simulink model "Fig1718"  (R2023b)
settings: Solver=ode1  StartTime=0.0  StopTime=32100  FixedStep=1  RelTol=1e-3
settings Model: Creator=orlandojorquera  LastModifiedBy=evogel

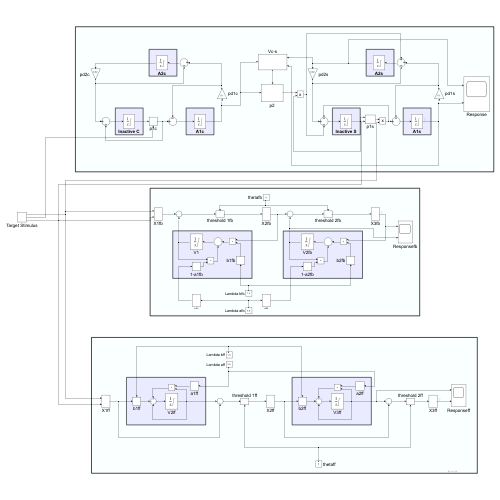
[thumbnail: Simulink's stored preview of the top-level diagram]
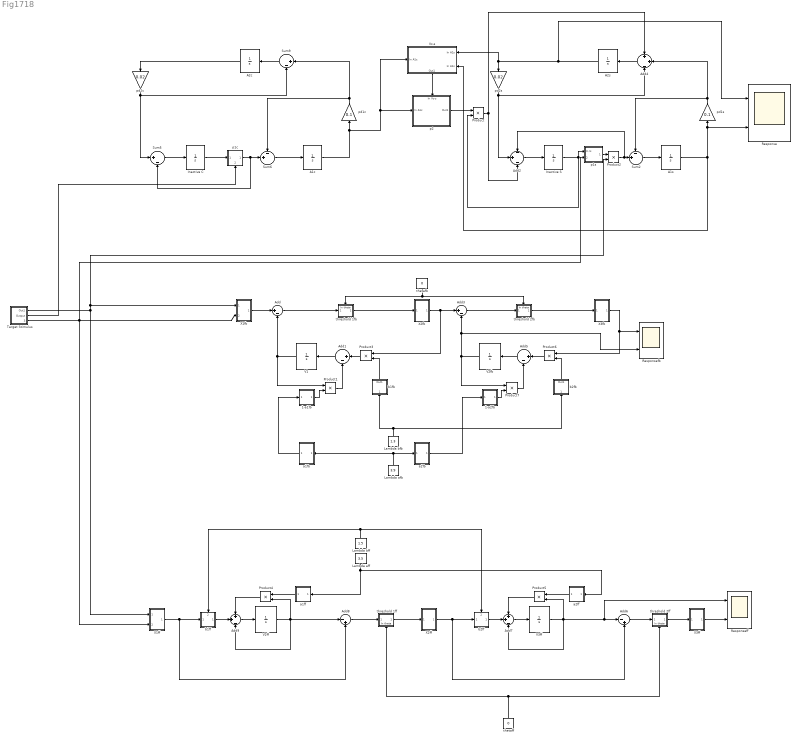
== system Fig1718 ==
  1-a1fb : Subsystem
  1-a2fb : Subsystem
  A1c : Integrator  LimitOutput=on  LowerSaturationLimit=0
  A1s : Integrator  LimitOutput=on  LowerSaturationLimit=0
  A2c : Integrator  LimitOutput=on  LowerSaturationLimit=0
  A2s : Integrator  LimitOutput=on  LowerSaturationLimit=0
  Add{,1,3,5} (4 alike) : Sum  Inputs=|+-
  Add2 : Sum  Inputs=-|+|-
  Add4 : Sum  Inputs=+|+|-
  Add6 : Sum  Inputs=|-+
  Add7 : Sum  Inputs=+|+|-
  Add8 : Sum  Inputs=|-+
  Add9 : Sum  Inputs=+|+|-
  Inactive C : Integrator  InitialCondition=1  LimitOutput=on  LowerSaturationLimit=0
  Inactive S : Integrator  InitialCondition=1  LimitOutput=on  LowerSaturationLimit=0
  Lambda afb : Constant  Value=3.9
  Lambda aff : Constant  Value=3.5
  Lambda bfb : Constant  Value=1.3
  Lambda bff : Constant  Value=1.5
  Product{,1..7} (8 alike) : Product
  Response : Scope  NumInputPorts=2
  Responsefb : Scope  NumInputPorts=2
  Responseff : Scope  NumInputPorts=2
  Sum2 : Sum  Inputs=-+|
  Sum5 : Sum  Inputs=|+-
  Sum6 : Sum  Inputs=-+|
  Sum9 : Sum  Inputs=|+-
  Target Stimulus : Subsystem
  V1 : Integrator  LimitOutput=on
  V2fb : Integrator  LimitOutput=on
  V2ff : Integrator  LimitOutput=on
  V3ff : Integrator  LimitOutput=on
  Vc-s : Subsystem
      settings: PortSchema="{\"entries\":[{\"content\":{\"sides\":[{\"content\":{\"connectorIds\":[\"In1\"]},\"type\":\"ConnectorPlacement.EquallySpacedRectSide\",\"uuid\":\"b09f05bd-5603-47fe-a5ad-d7d6b3dc0c8e\"},{\"content\":{\"connectorIds\":[\"In2\",\"In3\"],\"side\":\"RIGHT\"},\"type\":\"ConnectorPlacement.EquallySpacedRectSide\",\"uuid\":\"d47795f3-6d8c-4c23-a554-34b772022c1b\"},{\"content\":{\"side\":\"TOP\"},\"type\":\"ConnectorPlacement.EquallySpacedRectSide\",\"uuid\":\"e48eddfd-d331-425c-b357-ebbea553df38\"},{\"content\":{\"connectorIds\":[\"Out1\"],\"side\":\"BOTTOM\"},\"type\":\"ConnectorPlacement.EquallySpacedRectSide\",\"uuid\":\"833a9385-f8e7-4f69-9c09-473a519a1ef8\"}]},\"type\":\"ConnectorPlacement.EquallySpacedConnector\",\"uuid\":\"43dd1673-4710-4827-90f7-71f5e88827f7\"}],\"packageUris\":[\"http://schema.mathworks.com/mf0/Connector/R2020b\"],\"version\":\"1.0\"}"
  X1fb : Subsystem
  X1ff : Subsystem
  X2fb : Subsystem
  X2ff : Subsystem
  X3fb : Subsystem
  X3ff : Subsystem
  a1fb : Subsystem
  a1ff : Subsystem
  a2fb : Subsystem
  a2ff : Subsystem
  b1fb : Subsystem
  b1ff : Subsystem
      settings: PortSchema="{\"entries\":[{\"content\":{\"sides\":[{\"content\":{\"connectorIds\":[\"In1\"]},\"type\":\"ConnectorPlacement.EquallySpacedRectSide\",\"uuid\":\"5cafafed-fb19-4a9c-b5ff-e68617ed0211\"},{\"content\":{\"connectorIds\":[\"Out1\"],\"side\":\"RIGHT\"},\"type\":\"ConnectorPlacement.EquallySpacedRectSide\",\"uuid\":\"a77dc629-061a-4bf4-a80e-b7ca5c1ed4cd\"},{\"content\":{\"connectorIds\":[\"In2\"],\"side\":\"TOP\"},\"type\":\"ConnectorPlacement.EquallySpacedRectSide\",\"uuid\":\"07c5d7ad-6053-41a5-acdb-1c90061be6dc\"}]},\"type\":\"ConnectorPlacement.EquallySpacedConnector\",\"uuid\":\"79321a58-c601-4809-afd2-d30de13f135a\"}],\"packageUris\":[\"http://schema.mathworks.com/mf0/Connector/R2020b\"],\"version\":\"1.0\"}"
  b2fb : Subsystem
  b2ff : Subsystem
      settings: PortSchema="{\"entries\":[{\"content\":{\"sides\":[{\"content\":{\"connectorIds\":[\"In1\"]},\"type\":\"ConnectorPlacement.EquallySpacedRectSide\",\"uuid\":\"5cafafed-fb19-4a9c-b5ff-e68617ed0211\"},{\"content\":{\"connectorIds\":[\"Out1\"],\"side\":\"RIGHT\"},\"type\":\"ConnectorPlacement.EquallySpacedRectSide\",\"uuid\":\"a77dc629-061a-4bf4-a80e-b7ca5c1ed4cd\"},{\"content\":{\"connectorIds\":[\"In2\"],\"side\":\"TOP\"},\"type\":\"ConnectorPlacement.EquallySpacedRectSide\",\"uuid\":\"07c5d7ad-6053-41a5-acdb-1c90061be6dc\"}]},\"type\":\"ConnectorPlacement.EquallySpacedConnector\",\"uuid\":\"79321a58-c601-4809-afd2-d30de13f135a\"}],\"packageUris\":[\"http://schema.mathworks.com/mf0/Connector/R2020b\"],\"version\":\"1.0\"}"
  p1c : Subsystem
      settings: PortSchema="{\"entries\":[{\"content\":{\"sides\":[{\"content\":{\"connectorIds\":[\"In1\"]},\"type\":\"ConnectorPlacement.EquallySpacedRectSide\",\"uuid\":\"f7a9d23e-8fc7-4308-b994-1d41de704125\"},{\"content\":{\"connectorIds\":[\"Out1\"],\"side\":\"RIGHT\"},\"type\":\"ConnectorPlacement.EquallySpacedRectSide\",\"uuid\":\"dfc0205e-3a52-4ff6-ace9-e9ebe39396a1\"},{\"content\":{\"side\":\"TOP\"},\"type\":\"ConnectorPlacement.EquallySpacedRectSide\",\"uuid\":\"7914cb48-207a-4343-a956-bdfd7fe7ecdd\"},{\"content\":{\"connectorIds\":[\"In2\"],\"side\":\"BOTTOM\"},\"type\":\"ConnectorPlacement.EquallySpacedRectSide\",\"uuid\":\"56101731-0c9e-48a4-bdfd-b7c152720658\"}]},\"type\":\"ConnectorPlacement.EquallySpacedConnector\",\"uuid\":\"a86337d0-cbcf-4677-827f-1f8aa0c41de3\"}],\"packageUris\":[\"http://schema.mathworks.com/mf0/Connector/R2020b\"],\"version\":\"1.0\"}"
  p1s : Subsystem
  p2 : Subsystem
      settings: PortSchema="{\"entries\":[{\"content\":{\"sides\":[{\"content\":{\"connectorIds\":[\"In1\"]},\"type\":\"ConnectorPlacement.EquallySpacedRectSide\",\"uuid\":\"e5de33b1-e289-4f06-b16e-f6995d6ff18d\"},{\"content\":{\"connectorIds\":[\"Out1\"],\"side\":\"RIGHT\"},\"type\":\"ConnectorPlacement.EquallySpacedRectSide\",\"uuid\":\"bf82b542-ee2f-4a07-ac72-0e3e2437644b\"},{\"content\":{\"connectorIds\":[\"In2\"],\"side\":\"TOP\"},\"type\":\"ConnectorPlacement.EquallySpacedRectSide\",\"uuid\":\"dbd75b9a-fc8b-4088-9d34-f07ad0492047\"}]},\"type\":\"ConnectorPlacement.EquallySpacedConnector\",\"uuid\":\"24fb73df-5fe4-4caa-a2a9-0eaf37dbdd75\"}],\"packageUris\":[\"http://schema.mathworks.com/mf0/Connector/R2020b\"],\"version\":\"1.0\"}"
  pd1c : Gain  Gain=0.1
  pd1s : Gain  Gain=0.1
  pd2c : Gain  Gain=0.02
  pd2s : Gain  Gain=0.02
  thetafb : Constant  Value=0
  thetaff : Constant  Value=0
  threshold 1fb : Subsystem
      settings: PortSchema="{\"entries\":[{\"content\":{\"sides\":[{\"content\":{\"connectorIds\":[\"In1\"]},\"type\":\"ConnectorPlacement.EquallySpacedRectSide\",\"uuid\":\"df45c11a-cbfd-46b0-9931-ccf6bdc824b5\"},{\"content\":{\"connectorIds\":[\"Out1\"],\"side\":\"RIGHT\"},\"type\":\"ConnectorPlacement.EquallySpacedRectSide\",\"uuid\":\"7bdc14d3-84cb-4ad0-a730-e3b8f98cb716\"},{\"content\":{\"connectorIds\":[\"In2\"],\"side\":\"TOP\"},\"type\":\"ConnectorPlacement.EquallySpacedRectSide\",\"uuid\":\"6aa308ce-d9e8-4768-ab82-80fe1eba77b8\"}]},\"type\":\"ConnectorPlacement.EquallySpacedConnector\",\"uuid\":\"5c730a05-bfd2-4eaa-b46f-f4851af60a3b\"}],\"packageUris\":[\"http://schema.mathworks.com/mf0/Connector/R2020b\"],\"version\":\"1.0\"}"
  threshold 1ff : Subsystem
      settings: PortSchema="{\"entries\":[{\"content\":{\"sides\":[{\"content\":{\"connectorIds\":[\"In1\"]},\"type\":\"ConnectorPlacement.EquallySpacedRectSide\",\"uuid\":\"df45c11a-cbfd-46b0-9931-ccf6bdc824b5\"},{\"content\":{\"connectorIds\":[\"Out1\"],\"side\":\"RIGHT\"},\"type\":\"ConnectorPlacement.EquallySpacedRectSide\",\"uuid\":\"7bdc14d3-84cb-4ad0-a730-e3b8f98cb716\"},{\"content\":{\"side\":\"TOP\"},\"type\":\"ConnectorPlacement.EquallySpacedRectSide\",\"uuid\":\"6aa308ce-d9e8-4768-ab82-80fe1eba77b8\"},{\"content\":{\"connectorIds\":[\"In2\"],\"side\":\"BOTTOM\"},\"type\":\"ConnectorPlacement.EquallySpacedRectSide\",\"uuid\":\"e8fc9ce3-9b1c-421a-8c5e-f6ab306fc514\"}]},\"type\":\"ConnectorPlacement.EquallySpacedConnector\",\"uuid\":\"5c730a05-bfd2-4eaa-b46f-f4851af60a3b\"}],\"packageUris\":[\"http://schema.mathworks.com/mf0/Connector/R2020b\"],\"version\":\"1.0\"}"
  threshold 2fb : Subsystem
      settings: PortSchema="{\"entries\":[{\"content\":{\"sides\":[{\"content\":{\"connectorIds\":[\"In1\"]},\"type\":\"ConnectorPlacement.EquallySpacedRectSide\",\"uuid\":\"df45c11a-cbfd-46b0-9931-ccf6bdc824b5\"},{\"content\":{\"connectorIds\":[\"Out1\"],\"side\":\"RIGHT\"},\"type\":\"ConnectorPlacement.EquallySpacedRectSide\",\"uuid\":\"7bdc14d3-84cb-4ad0-a730-e3b8f98cb716\"},{\"content\":{\"connectorIds\":[\"In2\"],\"side\":\"TOP\"},\"type\":\"ConnectorPlacement.EquallySpacedRectSide\",\"uuid\":\"6aa308ce-d9e8-4768-ab82-80fe1eba77b8\"}]},\"type\":\"ConnectorPlacement.EquallySpacedConnector\",\"uuid\":\"5c730a05-bfd2-4eaa-b46f-f4851af60a3b\"}],\"packageUris\":[\"http://schema.mathworks.com/mf0/Connector/R2020b\"],\"version\":\"1.0\"}"
  threshold 2ff : Subsystem
      settings: PortSchema="{\"entries\":[{\"content\":{\"sides\":[{\"content\":{\"connectorIds\":[\"In1\"]},\"type\":\"ConnectorPlacement.EquallySpacedRectSide\",\"uuid\":\"df45c11a-cbfd-46b0-9931-ccf6bdc824b5\"},{\"content\":{\"connectorIds\":[\"Out1\"],\"side\":\"RIGHT\"},\"type\":\"ConnectorPlacement.EquallySpacedRectSide\",\"uuid\":\"7bdc14d3-84cb-4ad0-a730-e3b8f98cb716\"},{\"content\":{\"side\":\"TOP\"},\"type\":\"ConnectorPlacement.EquallySpacedRectSide\",\"uuid\":\"6aa308ce-d9e8-4768-ab82-80fe1eba77b8\"},{\"content\":{\"connectorIds\":[\"In2\"],\"side\":\"BOTTOM\"},\"type\":\"ConnectorPlacement.EquallySpacedRectSide\",\"uuid\":\"48b70d05-ed8a-416b-8c0e-25b0a2481944\"}]},\"type\":\"ConnectorPlacement.EquallySpacedConnector\",\"uuid\":\"5c730a05-bfd2-4eaa-b46f-f4851af60a3b\"}],\"packageUris\":[\"http://schema.mathworks.com/mf0/Connector/R2020b\"],\"version\":\"1.0\"}"
  wires:
  Inactive C/1 -> p1c/1(In1)
  Sum5/1 -> Inactive C/1
  p1c/1(Out1) -> Sum6/2, Sum5/2
  pd1c/1 -> Sum9/1, Sum6/1
  Sum6/1 -> A1c/1
  A1c/1 -> Vc-s/1(In A1c), p2/1(In A1c), pd1c/1
  Sum9/1 -> A2c/1
  A2c/1 -> pd2c/1
  pd2c/1 -> Sum5/1, Sum9/2
  Vc-s/1(Out1) -> p2/2(In Vc-s)
  pd2s/1 -> Add4/3, Add2/2
  A2s/1 -> Response/1, pd2s/1, Vc-s/2(In A2s)
  Add4/1 -> A2s/1
  A1s/1 -> Response/2, pd1s/1, Vc-s/3(In A1s)
  Sum2/1 -> A1s/1
  pd1s/1 -> Add4/2, Sum2/1
  Add2/1 -> Inactive S/1
  Inactive S/1 -> p1s/1(In Is), Product/2
  Product2/1 -> Add2/1, Sum2/2
  p2/1(Out1) -> Product/1
  Product/1 -> Add2/3, Add4/1
  1-a1fb/1(Out1) -> Product1/2
  Add3/1 -> threshold 2fb/1(In X2 - V2)
  Add/1 -> threshold 1fb/1(In X1 - V1)
  a1fb/1(Out1) -> 1-a1fb/1(In a1)
  X2fb/1(Out1) -> Product3/1, Add3/1
  1-a2fb/1(Out1) -> Product7/2
  X3fb/1(Out1) -> Product6/1, Responsefb/1
  V1/1 -> Product1/1, Add/2
  Add5/1 -> V2fb/1
  Product1/1 -> Add1/2
  V2fb/1 -> Add3/2, Responsefb/2, Product7/1
  threshold 2fb/1(Out1) -> X3fb/1(In1)
  Lambda bfb/1 -> b1fb/1(In lambda_b), b2fb/1(In lambda_b)
  Lambda afb/1 -> a1fb/1(In lambda_a), a2fb/1(In lambda_a)
  Add1/1 -> V1/1
  b2fb/1(Out1) -> Product6/2
  thetafb/1 -> threshold 1fb/2(In theta), threshold 2fb/2(In theta)
  a2fb/1(Out1) -> 1-a2fb/1(In a2)
  Product6/1 -> Add5/1
  b1fb/1(Out1) -> Product3/2
  threshold 1fb/1(Out1) -> X2fb/1(In1)
  Product3/1 -> Add1/1
  X1fb/1(Output) -> Add/1
  Product7/1 -> Add5/2
  ? -> ?
  thetaff/1 -> threshold 1ff/2(In theta), threshold 2ff/2(In theta)
  Add8/1 -> threshold 1ff/1(In X1 - V1)
  Product4/1 -> Add9/1
  X2ff/1(Output) -> Add6/2, b2ff/1(In1)
  threshold 1ff/1(Out1) -> X2ff/1(In Stimulus)
  b2ff/1(Out1) -> Add7/2
  V3ff/1 -> Product5/2, Responseff/1, Add6/1, Add7/3
  X3ff/1(Output) -> Responseff/2
  a1ff/1(Out1) -> Product4/1
  Add7/1 -> V3ff/1
  a2ff/1(Out1) -> Product5/1
  Add6/1 -> threshold 2ff/1(In X2 - V2)
  Target Stimulus/1(Out1) -> X1ff/1(In Stimulus), X1fb/1(In Stimulus), Product2/2
  V2ff/1 -> Add8/1, Product4/2, Add9/3
  Lambda aff/1 -> a2ff/1(In lambda_a), a1ff/1(In lambda_a)
  threshold 2ff/1(Out1) -> X3ff/1(In Stimulus)
  X1ff/1(Output) -> b1ff/1(In1), Add8/2
  Add9/1 -> V2ff/1
  Lambda bff/1 -> b1ff/2(In lambda_b), b2ff/2(In lambda_b)
  b1ff/1(Out1) -> Add9/2
  Product5/1 -> Add7/1
  Target Stimulus/2(Output) -> p1c/2(CTX on/off)
  Target Stimulus/3(Output1) -> p1s/2(In Intensity), X1ff/2(In Intensity), X1fb/2(In Intensity)
  p1s/1(Output) -> Product2/1

== system Fig1718/1-a1fb ==
  In a1 : Inport
  Add : Sum  Inputs=+-
  One : Constant  OutDataTypeStr=Inherit: Inherit via back propagation
  Out1 : Outport
  wires:
  One/1 -> Add/1
  Add/1 -> Out1/1
  In a1/1 -> Add/2

== system Fig1718/1-a2fb ==
  In a2 : Inport
  Add : Sum  Inputs=+-
  One : Constant  OutDataTypeStr=Inherit: Inherit via back propagation
  Out1 : Outport
  wires:
  In a2/1 -> Add/2
  Add/1 -> Out1/1
  One/1 -> Add/1

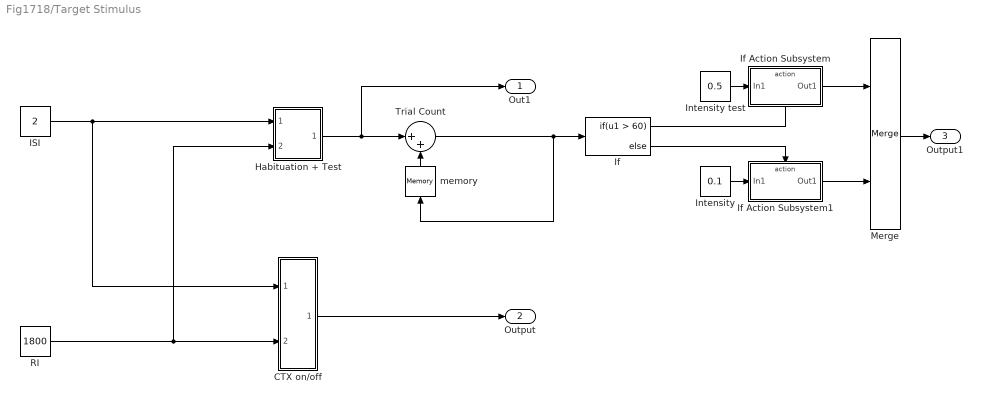
== system Fig1718/Target Stimulus ==
  CTX on/off : Subsystem
  Habituation + Test : Subsystem
  ISI : Constant  Value=2
  If : If  IfExpression=u1 > 60
  If Action Subsystem : Subsystem  TreatAsAtomicUnit=on
  If Action Subsystem1 : Subsystem  TreatAsAtomicUnit=on
  Intensity : Constant  Value=0.1
  Intensity test : Constant  Value=0.5
  Merge : Merge
  RI : Constant  Value=1800
  Trial Count : Sum  Inputs=|++
  memory : Memory
  Out1 : Outport
  Output : Outport  Port=2
  Output1 : Outport  Port=3
  wires:
  Habituation + Test/1(Out1) -> Out1/1, Trial Count/1
  memory/1 -> Trial Count/2
  Trial Count/1 -> If/1, memory/1
  RI/1 -> Habituation + Test/2(In RI), CTX on/off/2(In RI)
  CTX on/off/1(Output) -> Output/1
  If/1 -> If Action Subsystem/Action
  If/2 -> If Action Subsystem1/Action
  Intensity/1 -> If Action Subsystem1/1(In1)
  Intensity test/1 -> If Action Subsystem/1(In1)
  If Action Subsystem/1(Out1) -> Merge/1
  If Action Subsystem1/1(Out1) -> Merge/2
  Merge/1 -> Output1/1
  ISI/1 -> CTX on/off/1(In ISI), Habituation + Test/1(In ISI)

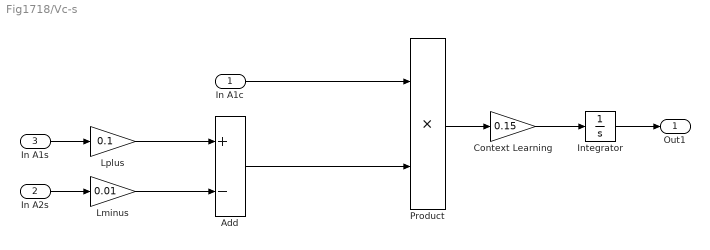
== system Fig1718/Vc-s ==
  In A1c : Inport
  In A2s : Inport  Port=2
  In A1s : Inport  Port=3
  Add : Sum  Inputs=+-
  Context Learning : Gain  Gain=0.15
  Integrator : Integrator  LimitOutput=on  LowerSaturationLimit=0
  Lminus : Gain  Gain=0.01
  Lplus : Gain  Gain=0.1
  Product : Product
  Out1 : Outport
  wires:
  In A1s/1 -> Lplus/1
  In A2s/1 -> Lminus/1
  In A1c/1 -> Product/1
  Product/1 -> Context Learning/1
  Context Learning/1 -> Integrator/1
  Add/1 -> Product/2
  Lplus/1 -> Add/1
  Lminus/1 -> Add/2
  Integrator/1 -> Out1/1

== system Fig1718/X1fb ==
  In Stimulus : Inport
  In Intensity : Inport  Port=2
  Product : Product
  Output : Outport
  wires:
  In Stimulus/1 -> Product/1
  Product/1 -> Output/1
  In Intensity/1 -> Product/2

== system Fig1718/X1ff ==
  In Stimulus : Inport
  In Intensity : Inport  Port=2
  Product : Product
  Output : Outport
  wires:
  In Intensity/1 -> Product/2
  Product/1 -> Output/1
  In Stimulus/1 -> Product/1

== system Fig1718/X2fb ==
  In1 : Inport
  Out1 : Outport
  wires:
  In1/1 -> Out1/1

== system Fig1718/X2ff ==
  In Stimulus : Inport
  Output : Outport
  wires:
  In Stimulus/1 -> Output/1

== system Fig1718/X3fb ==
  In1 : Inport
  Out1 : Outport
  wires:
  In1/1 -> Out1/1

== system Fig1718/X3ff ==
  In Stimulus : Inport
  Output : Outport
  wires:
  In Stimulus/1 -> Output/1

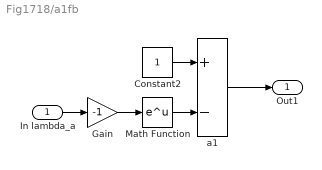
== system Fig1718/a1fb ==
  In lambda_a : Inport
  Constant2 : Constant
  Gain : Gain  Gain=-1
  Math Function : Math
  a1 : Sum  Inputs=+-
  Out1 : Outport
  wires:
  Math Function/1 -> a1/2
  Gain/1 -> Math Function/1
  Constant2/1 -> a1/1
  In lambda_a/1 -> Gain/1
  a1/1 -> Out1/1

== system Fig1718/a1ff ==
  In lambda_a : Inport
  Constant2 : Constant
  Gain : Gain  Gain=-1
  Math Function : Math
  a1 : Sum  Inputs=+-
  Out1 : Outport
  wires:
  Math Function/1 -> a1/2
  Gain/1 -> Math Function/1
  Constant2/1 -> a1/1
  In lambda_a/1 -> Gain/1
  a1/1 -> Out1/1

== system Fig1718/a2fb ==
  In lambda_a : Inport
  Constant2 : Constant
  Gain : Gain  Gain=-2
  Math Function : Math
  a1 : Sum  Inputs=+-
  Out1 : Outport
  wires:
  a1/1 -> Out1/1
  In lambda_a/1 -> Gain/1
  Constant2/1 -> a1/1
  Gain/1 -> Math Function/1
  Math Function/1 -> a1/2

== system Fig1718/a2ff ==
  In lambda_a : Inport
  Constant2 : Constant
  Gain : Gain  Gain=-2
  Math Function : Math
  a1 : Sum  Inputs=+-
  Out1 : Outport
  wires:
  a1/1 -> Out1/1
  In lambda_a/1 -> Gain/1
  Constant2/1 -> a1/1
  Gain/1 -> Math Function/1
  Math Function/1 -> a1/2

== system Fig1718/b1fb ==
  In lambda_b : Inport
  Gain : Gain  Gain=-1
  Math Function : Math
  Out1 : Outport
  wires:
  Math Function/1 -> Out1/1
  In lambda_b/1 -> Gain/1
  Gain/1 -> Math Function/1

== system Fig1718/b1ff ==
  In1 : Inport
  In lambda_b : Inport  Port=2
  Gain : Gain  Gain=-1
  Math Function : Math
  Product : Product
  Out1 : Outport
  wires:
  Gain/1 -> Math Function/1
  In lambda_b/1 -> Gain/1
  In1/1 -> Product/1
  Product/1 -> Out1/1
  Math Function/1 -> Product/2

== system Fig1718/b2fb ==
  In lambda_b : Inport
  Gain : Gain  Gain=-2
  Math Function : Math
  Out1 : Outport
  wires:
  Gain/1 -> Math Function/1
  In lambda_b/1 -> Gain/1
  Math Function/1 -> Out1/1

== system Fig1718/b2ff ==
  In1 : Inport
  In lambda_b : Inport  Port=2
  Gain : Gain  Gain=-2
  Math Function : Math
  Product : Product
  Out1 : Outport
  wires:
  Math Function/1 -> Product/2
  Product/1 -> Out1/1
  In1/1 -> Product/1
  In lambda_b/1 -> Gain/1
  Gain/1 -> Math Function/1

== system Fig1718/p1c ==
  In1 : Inport
  CTX on/off : Inport  Port=2
  Gain : Gain  Gain=0.05
  Product : Product
  Out1 : Outport
  wires:
  Gain/1 -> Out1/1
  Product/1 -> Gain/1
  In1/1 -> Product/1
  CTX on/off/1 -> Product/2

== system Fig1718/p1s ==
  In Is : Inport
  In Intensity : Inport  Port=2
  Product : Product
  Output : Outport
  wires:
  In Intensity/1 -> Product/2
  In Is/1 -> Product/1
  Product/1 -> Output/1

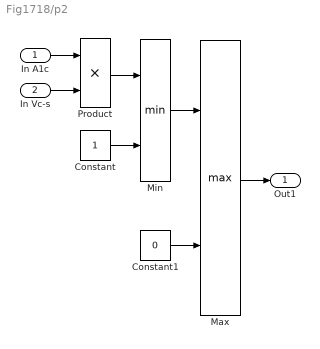
== system Fig1718/p2 ==
  In A1c : Inport
  In Vc-s : Inport  Port=2
  Constant : Constant
  Constant1 : Constant  Value=0
  Max : MinMax  Function=max  Inputs=2
  Min : MinMax  Inputs=2
  Product : Product
  Out1 : Outport
  wires:
  In Vc-s/1 -> Product/2
  In A1c/1 -> Product/1
  Product/1 -> Min/1
  Constant/1 -> Min/2
  Min/1 -> Max/1
  Constant1/1 -> Max/2
  Max/1 -> Out1/1

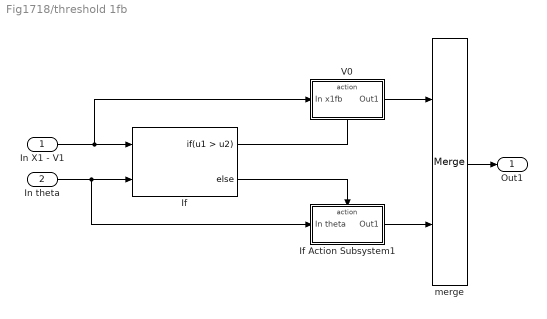
== system Fig1718/threshold 1fb ==
  In X1 - V1 : Inport
  In theta : Inport  Port=2
  If : If  NumInputs=2  IfExpression=u1 > u2
  If Action Subsystem1 : Subsystem  TreatAsAtomicUnit=on
  V0 : Subsystem  TreatAsAtomicUnit=on
  merge : Merge
  Out1 : Outport
  wires:
  V0/1(Out1) -> merge/1
  merge/1 -> Out1/1
  If Action Subsystem1/1(Out1) -> merge/2
  In theta/1 -> If Action Subsystem1/1(In theta), If/2
  In X1 - V1/1 -> V0/1(In x1fb), If/1
  If/1 -> V0/Action
  If/2 -> If Action Subsystem1/Action

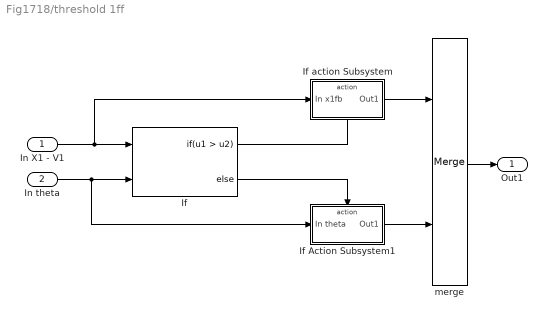
== system Fig1718/threshold 1ff ==
  In X1 - V1 : Inport
  In theta : Inport  Port=2
  If : If  NumInputs=2  IfExpression=u1 > u2
  If Action Subsystem1 : Subsystem  TreatAsAtomicUnit=on
  If action Subsystem : Subsystem  TreatAsAtomicUnit=on
  merge : Merge
  Out1 : Outport
  wires:
  If/2 -> If Action Subsystem1/Action
  If/1 -> If action Subsystem/Action
  In X1 - V1/1 -> If/1, If action Subsystem/1(In x1fb)
  In theta/1 -> If/2, If Action Subsystem1/1(In theta)
  If Action Subsystem1/1(Out1) -> merge/2
  merge/1 -> Out1/1
  If action Subsystem/1(Out1) -> merge/1

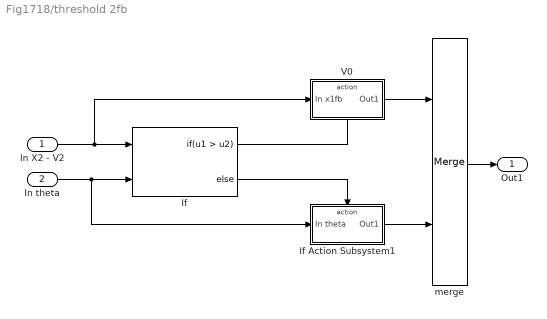
== system Fig1718/threshold 2fb ==
  In X2 - V2 : Inport
  In theta : Inport  Port=2
  If : If  NumInputs=2  IfExpression=u1 > u2
  If Action Subsystem1 : Subsystem  TreatAsAtomicUnit=on
  V0 : Subsystem  TreatAsAtomicUnit=on
  merge : Merge
  Out1 : Outport
  wires:
  If/2 -> If Action Subsystem1/Action
  If/1 -> V0/Action
  In X2 - V2/1 -> If/1, V0/1(In x1fb)
  In theta/1 -> If/2, If Action Subsystem1/1(In theta)
  If Action Subsystem1/1(Out1) -> merge/2
  merge/1 -> Out1/1
  V0/1(Out1) -> merge/1

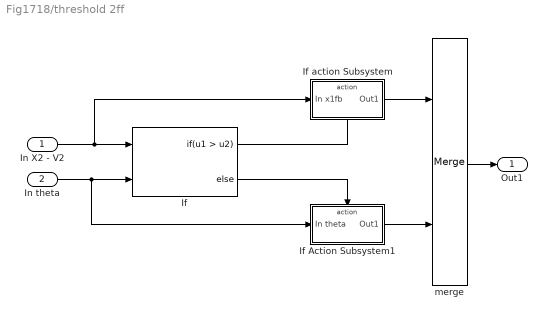
== system Fig1718/threshold 2ff ==
  In X2 - V2 : Inport
  In theta : Inport  Port=2
  If : If  NumInputs=2  IfExpression=u1 > u2
  If Action Subsystem1 : Subsystem  TreatAsAtomicUnit=on
  If action Subsystem : Subsystem  TreatAsAtomicUnit=on
  merge : Merge
  Out1 : Outport
  wires:
  If action Subsystem/1(Out1) -> merge/1
  merge/1 -> Out1/1
  If Action Subsystem1/1(Out1) -> merge/2
  In theta/1 -> If Action Subsystem1/1(In theta), If/2
  In X2 - V2/1 -> If action Subsystem/1(In x1fb), If/1
  If/1 -> If action Subsystem/Action
  If/2 -> If Action Subsystem1/Action

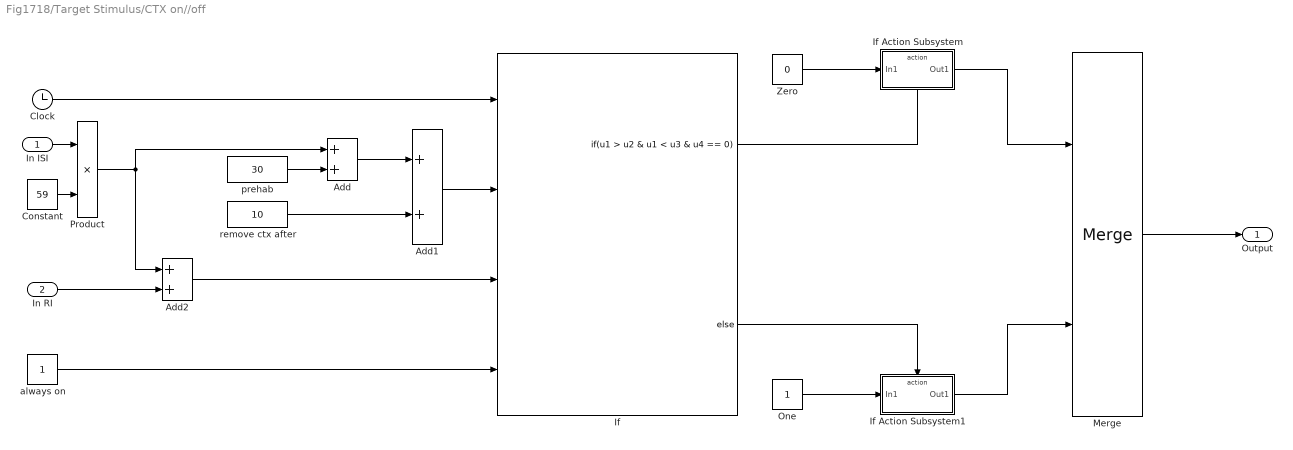
== system Fig1718/Target Stimulus/CTX on//off ==
  In ISI : Inport
  In RI : Inport  Port=2
  " prehab" : Constant  Value=30
  " remove ctx after " : Constant  Value=10
  Add : Sum
  Add1 : Sum
  Add2 : Sum
  Clock : Clock
  Constant : Constant  Value=59
  If : If  NumInputs=4  IfExpression=u1 > u2 & u1 < u3 & u4 == 0
  If Action Subsystem : Subsystem  TreatAsAtomicUnit=on
  If Action Subsystem1 : Subsystem  TreatAsAtomicUnit=on
  Merge : Merge
  One : Constant  OutDataTypeStr=Inherit: Inherit via back propagation
  Product : Product
  Zero : Constant  Value=0  OutDataTypeStr=Inherit: Inherit via back propagation
  always on : Constant
  Output : Outport
  wires:
  Constant/1 -> Product/2
  Clock/1 -> If/1
  In RI/1 -> Add2/2
  Product/1 -> Add/1, Add2/1
  " prehab"/1 -> Add/2
  Add/1 -> Add1/1
  If/1 -> If Action Subsystem/Action
  Zero/1 -> If Action Subsystem/1(In1)
  If/2 -> If Action Subsystem1/Action
  One/1 -> If Action Subsystem1/1(In1)
  If Action Subsystem/1(Out1) -> Merge/1
  If Action Subsystem1/1(Out1) -> Merge/2
  Merge/1 -> Output/1
  " remove ctx after "/1 -> Add1/2
  Add1/1 -> If/2
  Add2/1 -> If/3
  always on/1 -> If/4
  In ISI/1 -> Product/1

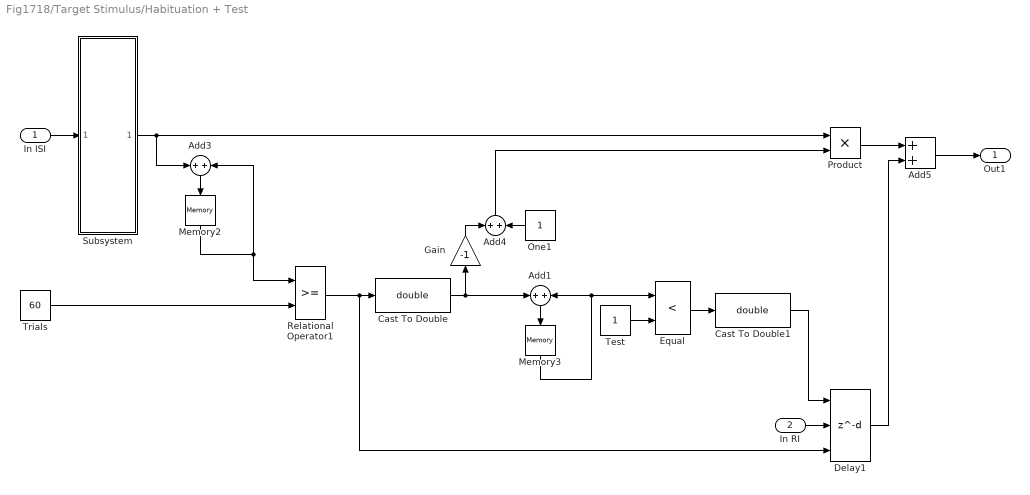
== system Fig1718/Target Stimulus/Habituation + Test ==
  In ISI : Inport
  In RI : Inport  Port=2
  Add{1,3..5} (4 alike) : Sum
  Cast To Double : DataTypeConversion  OutDataTypeStr=double  SaturateOnIntegerOverflow=off  RndMeth=Floor
  Cast To Double1 : DataTypeConversion  OutDataTypeStr=double  SaturateOnIntegerOverflow=off  RndMeth=Floor
  Delay1 : Delay  DelayLengthSource=Input port  DelayLength=250  DelayLengthUpperLimit=4000  ShowEnablePort=on
      settings: InputPortMap=u0,p1,e6
  Equal : RelationalOperator  Operator=<  OutDataTypeStr=boolean  RndMeth=Simplest  InputSameDT=off
  Gain : Gain  Gain=-1
  Memory2 : Memory
  Memory3 : Memory
  One1 : Constant  OutDataTypeStr=Inherit: Inherit via back propagation
  Product : Product
  Relational Operator1 : RelationalOperator  OutDataTypeStr=boolean  RndMeth=Simplest  InputSameDT=off
  Subsystem : Subsystem
  Test : Constant  OutDataTypeStr=Inherit: Inherit via back propagation
  Trials : Constant  Value=60
  Out1 : Outport
  wires:
  Subsystem/1(Out2) -> Add3/1, Product/1
  Add3/1 -> Memory2/1
  Memory2/1 -> Relational Operator1/1, Add3/2
  Trials/1 -> Relational Operator1/2
  Relational Operator1/1 -> Delay1/3, Cast To Double/1
  Cast To Double/1 -> Gain/1, Add1/1
  Add1/1 -> Memory3/1
  Memory3/1 -> Add1/2, Equal/1
  Test/1 -> Equal/2
  Equal/1 -> Cast To Double1/1
  Gain/1 -> Add4/1
  One1/1 -> Add4/2
  Add4/1 -> Product/2
  Cast To Double1/1 -> Delay1/1
  Product/1 -> Add5/1
  Delay1/1 -> Add5/2
  Add5/1 -> Out1/1
  In RI/1 -> Delay1/2
  In ISI/1 -> Subsystem/1(In ISI)

== system Fig1718/Target Stimulus/If Action Subsystem ==
  In1 : Inport
  Action Port : ActionPort  ActionPortLabel=if(u1 > 60)
  Out1 : Outport
  wires:
  In1/1 -> Out1/1

== system Fig1718/Target Stimulus/If Action Subsystem1 ==
  In1 : Inport
  Action Port : ActionPort  ActionPortLabel=else
  Out1 : Outport
  wires:
  In1/1 -> Out1/1

== system Fig1718/threshold 1fb/If Action Subsystem1 ==
  In theta : Inport
  Action Port : ActionPort  ActionPortLabel=else
  Out1 : Outport
  wires:
  In theta/1 -> Out1/1

== system Fig1718/threshold 1fb/V0 ==
  In x1fb : Inport
  Action Port : ActionPort  ActionPortLabel=if(u1 > u2)
  Out1 : Outport
  wires:
  In x1fb/1 -> Out1/1

== system Fig1718/threshold 1ff/If Action Subsystem1 ==
  In theta : Inport
  Action Port : ActionPort  ActionPortLabel=else
  Out1 : Outport
  wires:
  In theta/1 -> Out1/1

== system Fig1718/threshold 1ff/If action Subsystem ==
  In x1fb : Inport
  Action Port : ActionPort  ActionPortLabel=if(u1 > u2)
  Out1 : Outport
  wires:
  In x1fb/1 -> Out1/1

== system Fig1718/threshold 2fb/If Action Subsystem1 ==
  In theta : Inport
  Action Port : ActionPort  ActionPortLabel=else
  Out1 : Outport
  wires:
  In theta/1 -> Out1/1

== system Fig1718/threshold 2fb/V0 ==
  In x1fb : Inport
  Action Port : ActionPort  ActionPortLabel=if(u1 > u2)
  Out1 : Outport
  wires:
  In x1fb/1 -> Out1/1

== system Fig1718/threshold 2ff/If Action Subsystem1 ==
  In theta : Inport
  Action Port : ActionPort  ActionPortLabel=else
  Out1 : Outport
  wires:
  In theta/1 -> Out1/1

== system Fig1718/threshold 2ff/If action Subsystem ==
  In x1fb : Inport
  Action Port : ActionPort  ActionPortLabel=if(u1 > u2)
  Out1 : Outport
  wires:
  In x1fb/1 -> Out1/1

== system Fig1718/Target Stimulus/CTX on//off/If Action Subsystem ==
  In1 : Inport
  Action Port : ActionPort  ActionPortLabel=if(u1 > u2 & u1 < u3 & u4 == 0)
  Out1 : Outport
  wires:
  In1/1 -> Out1/1

== system Fig1718/Target Stimulus/CTX on//off/If Action Subsystem1 ==
  In1 : Inport
  Action Port : ActionPort  ActionPortLabel=else
  Out1 : Outport
  wires:
  In1/1 -> Out1/1

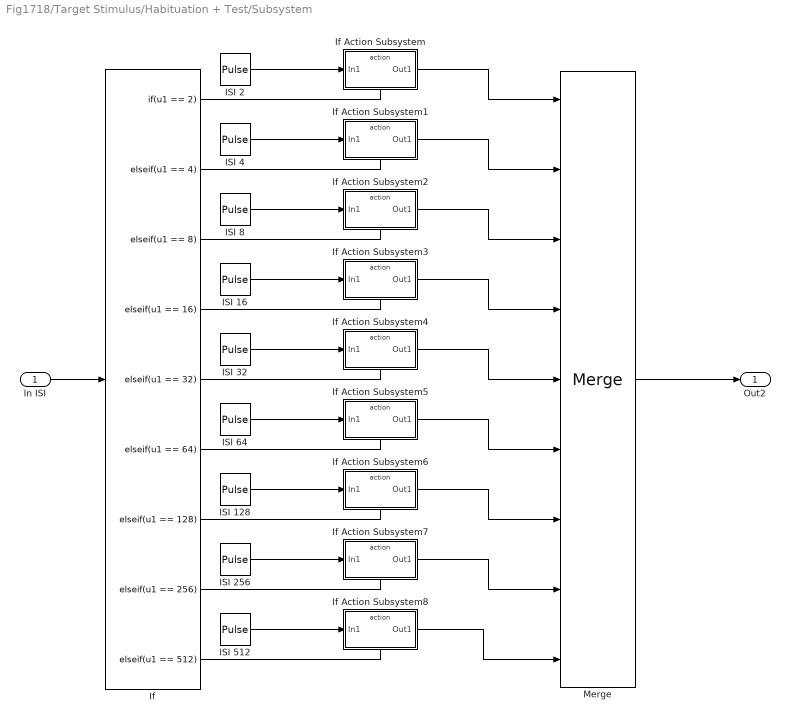
== system Fig1718/Target Stimulus/Habituation + Test/Subsystem ==
  In ISI : Inport
  ISI 128 : DiscretePulseGenerator  Period=128  PhaseDelay=30
  ISI 16 : DiscretePulseGenerator  Period=16  PhaseDelay=30
  ISI 2 : DiscretePulseGenerator  PhaseDelay=30
  ISI 256 : DiscretePulseGenerator  Period=256  PhaseDelay=30
  ISI 32 : DiscretePulseGenerator  Period=32  PhaseDelay=30
  ISI 4 : DiscretePulseGenerator  Period=4  PhaseDelay=30
  ISI 512 : DiscretePulseGenerator  Period=512  PhaseDelay=30
  ISI 64 : DiscretePulseGenerator  Period=64  PhaseDelay=30
  ISI 8 : DiscretePulseGenerator  Period=8  PhaseDelay=30
  If : If  IfExpression=u1 == 2  ElseIfExpressions=u1 == 4, u1 == 8, u1 == 16, u1 == 32, u1 == 64, u1 == 128, u1 == 256, u1 == 512  ShowElse=off
  If Action Subsystem : Subsystem  TreatAsAtomicUnit=on
  If Action Subsystem1 : Subsystem  TreatAsAtomicUnit=on
  If Action Subsystem2 : Subsystem  TreatAsAtomicUnit=on
  If Action Subsystem3 : Subsystem  TreatAsAtomicUnit=on
  If Action Subsystem4 : Subsystem  TreatAsAtomicUnit=on
  If Action Subsystem5 : Subsystem  TreatAsAtomicUnit=on
  If Action Subsystem6 : Subsystem  TreatAsAtomicUnit=on
  If Action Subsystem7 : Subsystem  TreatAsAtomicUnit=on
  If Action Subsystem8 : Subsystem  TreatAsAtomicUnit=on
  Merge : Merge  Inputs=9
  Out2 : Outport
  wires:
  ISI 2/1 -> If Action Subsystem/1(In1)
  In ISI/1 -> If/1
  If/1 -> If Action Subsystem/Action
  If/2 -> If Action Subsystem1/Action
  If/3 -> If Action Subsystem2/Action
  If/4 -> If Action Subsystem3/Action
  If/5 -> If Action Subsystem4/Action
  If/9 -> If Action Subsystem8/Action
  If/8 -> If Action Subsystem7/Action
  If/7 -> If Action Subsystem6/Action
  If/6 -> If Action Subsystem5/Action
  ISI 4/1 -> If Action Subsystem1/1(In1)
  ISI 8/1 -> If Action Subsystem2/1(In1)
  ISI 16/1 -> If Action Subsystem3/1(In1)
  ISI 32/1 -> If Action Subsystem4/1(In1)
  ISI 64/1 -> If Action Subsystem5/1(In1)
  ISI 128/1 -> If Action Subsystem6/1(In1)
  ISI 256/1 -> If Action Subsystem7/1(In1)
  ISI 512/1 -> If Action Subsystem8/1(In1)
  If Action Subsystem8/1(Out1) -> Merge/9
  If Action Subsystem7/1(Out1) -> Merge/8
  If Action Subsystem6/1(Out1) -> Merge/7
  If Action Subsystem5/1(Out1) -> Merge/6
  If Action Subsystem4/1(Out1) -> Merge/5
  If Action Subsystem3/1(Out1) -> Merge/4
  If Action Subsystem2/1(Out1) -> Merge/3
  If Action Subsystem1/1(Out1) -> Merge/2
  If Action Subsystem/1(Out1) -> Merge/1
  Merge/1 -> Out2/1

== system Fig1718/Target Stimulus/Habituation + Test/Subsystem/If Action Subsystem ==
  In1 : Inport
  Action Port : ActionPort  ActionPortLabel=if(u1 == 2)
  Out1 : Outport
  wires:
  In1/1 -> Out1/1

== system Fig1718/Target Stimulus/Habituation + Test/Subsystem/If Action Subsystem1 ==
  In1 : Inport
  Action Port : ActionPort  ActionPortLabel=elseif(u1 == 4)
  Out1 : Outport
  wires:
  In1/1 -> Out1/1

== system Fig1718/Target Stimulus/Habituation + Test/Subsystem/If Action Subsystem2 ==
  In1 : Inport
  Action Port : ActionPort  ActionPortLabel=elseif( u1 == 8)
  Out1 : Outport
  wires:
  In1/1 -> Out1/1

== system Fig1718/Target Stimulus/Habituation + Test/Subsystem/If Action Subsystem3 ==
  In1 : Inport
  Action Port : ActionPort  ActionPortLabel=elseif( u1 == 16)
  Out1 : Outport
  wires:
  In1/1 -> Out1/1

== system Fig1718/Target Stimulus/Habituation + Test/Subsystem/If Action Subsystem4 ==
  In1 : Inport
  Action Port : ActionPort  ActionPortLabel=elseif( u1 == 32)
  Out1 : Outport
  wires:
  In1/1 -> Out1/1

== system Fig1718/Target Stimulus/Habituation + Test/Subsystem/If Action Subsystem5 ==
  In1 : Inport
  Action Port : ActionPort  ActionPortLabel=elseif( u1 == 64)
  Out1 : Outport
  wires:
  In1/1 -> Out1/1

== system Fig1718/Target Stimulus/Habituation + Test/Subsystem/If Action Subsystem6 ==
  In1 : Inport
  Action Port : ActionPort  ActionPortLabel=elseif( u1 == 128)
  Out1 : Outport
  wires:
  In1/1 -> Out1/1

== system Fig1718/Target Stimulus/Habituation + Test/Subsystem/If Action Subsystem7 ==
  In1 : Inport
  Action Port : ActionPort  ActionPortLabel=elseif( u1 == 256)
  Out1 : Outport
  wires:
  In1/1 -> Out1/1

== system Fig1718/Target Stimulus/Habituation + Test/Subsystem/If Action Subsystem8 ==
  In1 : Inport
  Action Port : ActionPort  ActionPortLabel=elseif( u1 == 512)
  Out1 : Outport
  wires:
  In1/1 -> Out1/1
